simulink model "mechanicalSystmes"  (R2021a)
settings: Solver=VariableStepAuto  StartTime=0.0  StopTime=10  FixedStep=0.001  RelTol=1e-3
model workspace (MAT data in the model file):
  b = Simulink.Parameter
  b.Value = 1
  b.DataType = 'int8'
  b.Dimensions = [1 1]
  m = Simulink.Parameter
  m.Value = 1
  m.DataType = 'int8'
  m.Dimensions = [1 1]
undefined symbols (not defined in the file): k
settings Model: OrderedModelArguments=off  Creator=User  LastModifiedBy=User
settings OptimizationCC: DefaultParameterBehavior=Inlined  EnhancedBackFolding=on  PassReuseOutputArgsAs=Individual arguments  ZeroExternalMemoryAtStartup=off  ZeroInternalMemoryAtStartup=off  OptimizeBlockOrder=speed  DifferentSizesBufferReuse=on  OptimizationCustomize=off  EfficientTunableParamExpr=on
settings DebuggingCC: ParameterTunabilityLossMsg=error
settings SFSimCC: MATLABDynamicMemAlloc=off
settings RTWCC: SystemTargetFile=ert.tlc  TemplateMakefile=ert_default_tmf
settings CodeAppCC: ForceParamTrailComments=on  IgnoreCustomStorageClasses=off  OperatorAnnotations=on  SimulinkDataObjDesc=on  SFDataObjDesc=on  InsertBlockDesc=on
settings ERTTargetCC: TargetLangStandard=C99 (ISO)  GenerateSampleERTMain=on  InlinedParameterPlacement=NonHierarchical  ERTCustomFileTemplate=example_file_process.tlc
settings ConfigComp: CovScope=ReferencedModels  CovIncludeTopModel=off  CovMetricSettings=dcmwe

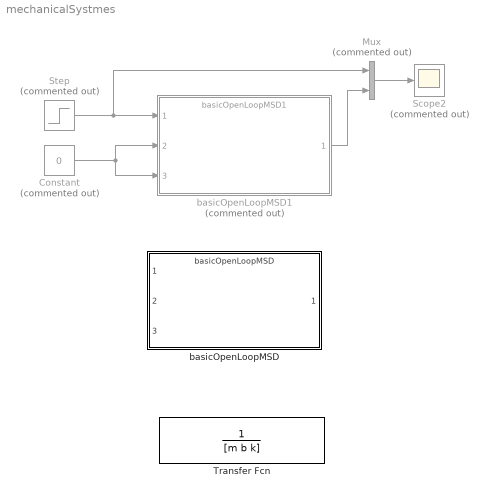
== system mechanicalSystmes ==
  Constant : Constant  Commented=on  Value=0
  Mux : Mux  Commented=on  Inputs=2
  Scope2 : Scope  Commented=on
  Step : Step  Commented=on  SampleTime=0
  Transfer Fcn : TransferFcn  Denominator=[m b k]
  basicOpenLoopMSD : ModelReference  ModelNameDialog=basicOpenLoopMSD  SimulationMode=Software-in-the-loop (SIL)  ModelReferenceVersion=1.10
  basicOpenLoopMSD1 : ModelReference  Commented=on  ModelNameDialog=basicOpenLoopMSD1  SimulationMode=Normal  ModelReferenceVersion=1.9
  wires:
  Mux/1 -> Scope2/1
  basicOpenLoopMSD1/1 -> Mux/2
  Step/1 -> Mux/1, basicOpenLoopMSD1/1
  Constant/1 -> basicOpenLoopMSD1/3, basicOpenLoopMSD1/2
